simulink model "Vehicle_Performance"  (R2016a)
settings: Solver=ode23s  StartTime=0.0  StopTime=12  FixedStep=0.1  RelTol=1e-3
values from neighbouring files (symbols this model uses):
  a = 0.84    [Vehicle_Performance.mat]
  c = 3100    [Vehicle_Performance.mat]
  d = 30    [Vehicle_Performance.mat]    (also in car_suspension.mat = 0.348888888889)
  e = 2    [Vehicle_Performance.mat]
  gb = 10    [Vehicle_Performance.mat]
  h = 0.65    [Vehicle_Performance.mat]    (also in car_suspension.mat = 353)
  hgr = 0.9    [Vehicle_Performance.mat]
  l = 1.3    [Vehicle_Performance.mat]
  lgr = 3.9    [Vehicle_Performance.mat]
  m = 210    [Vehicle_Performance.mat]
  o = 0    [Vehicle_Performance.mat]
  r = 0.2794    [Vehicle_Performance.mat]    (also in car_suspension.mat = 279.4)
libraries: simulink x3
settings Model: Creator=Lenovo  LastModifiedBy=admin
settings SolverCC: MaxConsecutiveMinStep=100
settings DataIOCC: LimitDataPoints=on  SaveFormat=Array
settings DebuggingCC: AlgebraicLoopMsg=none  ArtificialAlgebraicLoopMsg=none  ParameterPrecisionLossMsg=none
settings HardwareCC: ProdBitPerPointer=32  ProdLargestAtomicFloat=None  ProdIntDivRoundTo=Undefined  ProdEndianess=Unspecified  ProdWordSize=32  ProdHWDeviceType=32-bit Generic
settings ModelReferenceCC: PropagateSignalLabelsOutOfModel=off
settings ConfigComp: CovModelRefEnable=Off  CovSFcnEnable=off
settings ConfigurationSet: Description=SimMechanics 2G

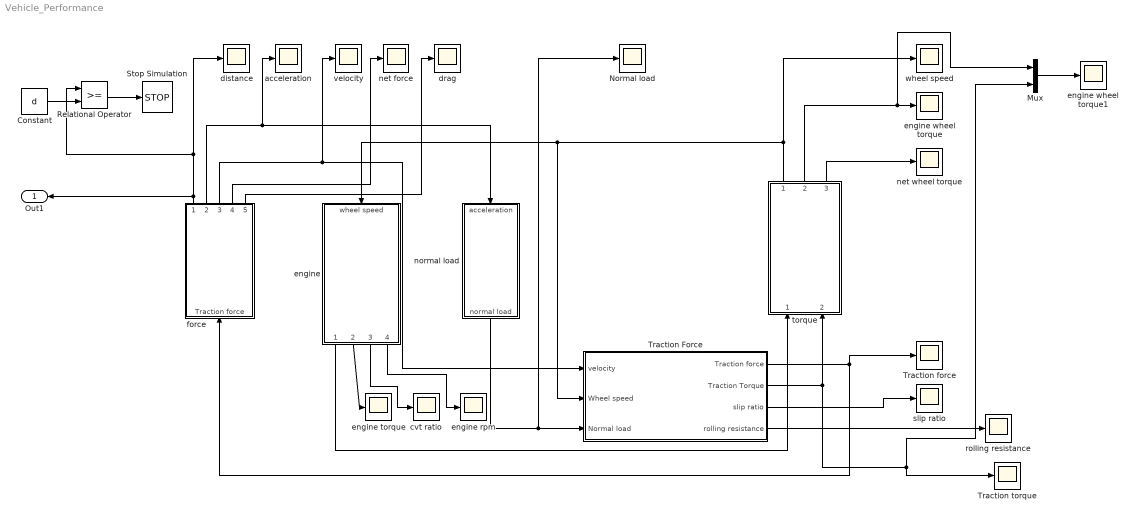
== system Vehicle_Performance ==
  Constant : Constant  Value=d
  Mux : Mux  Inputs=2
  Normal load : Scope
  Relational Operator : RelationalOperator  OutDataTypeStr=boolean
  Stop Simulation : Stop
  Traction Force : Subsystem
  Traction force : Scope
  Traction torque : Scope
  acceleration : Scope
  cvt ratio : Scope
  distance : Scope
  drag : Scope
  "engine " : Subsystem
  engine rpm : Scope
  engine torque : Scope
  engine wheel torque : Scope
  engine wheel torque1 : Scope
  force : Subsystem
  net force : Scope
  net wheel torque : Scope
  normal load : Subsystem
  rolling resistance : Scope
  slip ratio : Scope
  torque : Subsystem
  "velocity " : Scope
  "wheel speed " : Scope
  Out1 : Outport
  wires:
  "engine "/1("wheel torque ") -> torque/1(Wheel torque)
  torque/1("wheel speed ") -> "engine "/1("wheel speed "), Traction Force/2(Wheel speed), "wheel speed "/1
  force/2(acceleration) -> normal load/1(acceleration), acceleration/1
  force/3(Velocity) -> "velocity "/1, Traction Force/1(velocity)
  normal load/1("normal load ") -> Normal load/1, Traction Force/3(Normal load)
  Traction Force/1(Traction force) -> Traction force/1, force/1(Traction force)
  force/1(distance) -> Relational Operator/1, distance/1, Out1/1
  Traction Force/3(slip ratio) -> slip ratio/1
  Traction Force/2(Traction Torque) -> torque/2(Traction torque), Mux/2, Traction torque/1
  torque/3(net wheel torque) -> net wheel torque/1
  force/4(net force) -> net force/1
  force/5(drag force) -> drag/1
  Traction Force/4(rolling resistance) -> rolling resistance/1
  Constant/1 -> Relational Operator/2
  Relational Operator/1 -> Stop Simulation/1
  torque/2(engine wheel torque) -> Mux/1, engine wheel torque/1
  "engine "/2("engine torque  ") -> engine torque/1
  Mux/1 -> engine wheel torque1/1
  "engine "/3(cvt ratio) -> cvt ratio/1
  "engine "/4(engine rpm) -> engine rpm/1

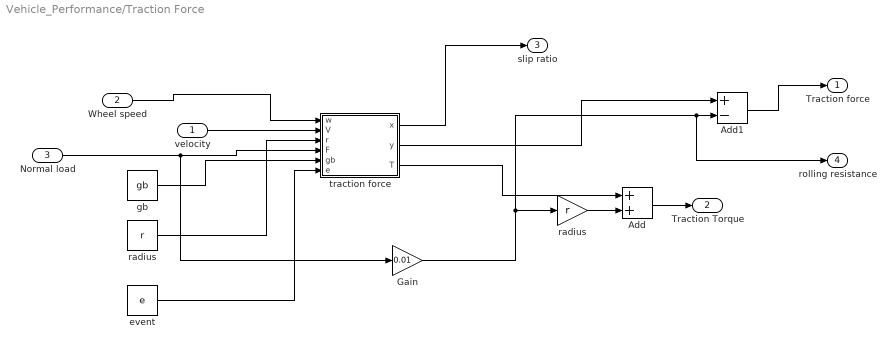
== system Vehicle_Performance/Traction Force ==
  velocity : Inport
  Wheel speed : Inport  Port=2
  Normal load : Inport  Port=3
  Add : Sum
  Add1 : Sum  Inputs=+-
  Gain : Gain  Gain=0.01
  event : Constant  Value=e
  "gb " : Constant  Value=gb
  radius : Gain  Gain=r
  "radius " : Constant  Value=r
  "traction force " : MATLAB Function  TreatAsAtomicUnit=on
  Traction force : Outport
  Traction Torque : Outport  Port=2
  slip ratio : Outport  Port=3
  rolling resistance : Outport  Port=4
  wires:
  velocity/1 -> "traction force "/2(V)
  Wheel speed/1 -> "traction force "/1(w)
  "gb "/1 -> "traction force "/5(gb)
  Normal load/1 -> "traction force "/4(F), Gain/1
  "traction force "/1(x) -> slip ratio/1
  Add/1 -> Traction Torque/1
  "traction force "/3(T) -> Add/1
  Gain/1 -> radius/1, rolling resistance/1, Add1/2
  Add1/1 -> Traction force/1
  "traction force "/2(y) -> Add1/1
  radius/1 -> Add/2
  "radius "/1 -> "traction force "/3(r)
  event/1 -> "traction force "/6(e)

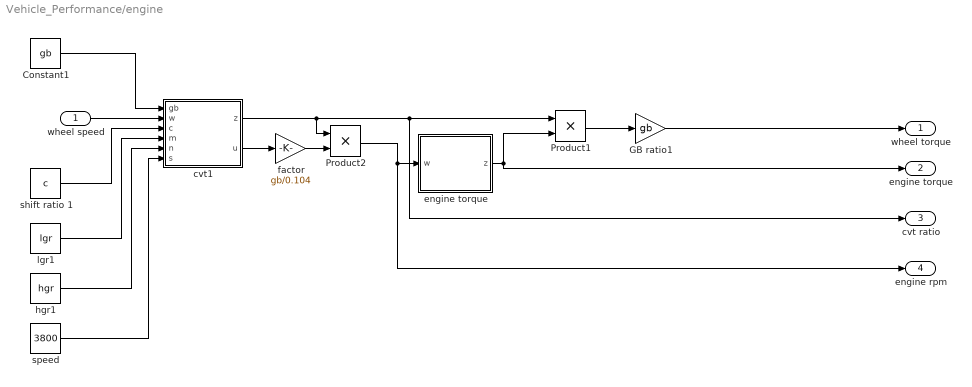
== system Vehicle_Performance/engine  ==
  "wheel speed " : Inport
  Constant1 : Constant  Value=gb
  GB ratio1 : Gain  Gain=gb
  Product1 : Product
  Product2 : Product
  cvt1 : MATLAB Function  TreatAsAtomicUnit=on
  engine torque : MATLAB Function  TreatAsAtomicUnit=on
  factor : Gain  Gain=gb/0.104
  hgr1 : Constant  Value=hgr
  lgr1 : Constant  Value=lgr
  shift ratio 1 : Constant  Value=c
  speed : Constant  Value=3800
  "wheel torque " : Outport
  "engine torque  " : Outport  Port=2
  cvt ratio : Outport  Port=3
  engine rpm : Outport  Port=4
  wires:
  Product1/1 -> GB ratio1/1
  engine torque/1(z) -> "engine torque  "/1, Product1/2
  cvt1/1(z) -> cvt ratio/1, Product1/1, Product2/1
  cvt1/2(u) -> factor/1
  factor/1 -> Product2/2
  Constant1/1 -> cvt1/1(gb)
  shift ratio 1/1 -> cvt1/3(c)
  lgr1/1 -> cvt1/4(m)
  hgr1/1 -> cvt1/5(n)
  speed/1 -> cvt1/6(s)
  Product2/1 -> engine rpm/1, engine torque/1(w)
  GB ratio1/1 -> "wheel torque "/1
  "wheel speed "/1 -> cvt1/2(w)

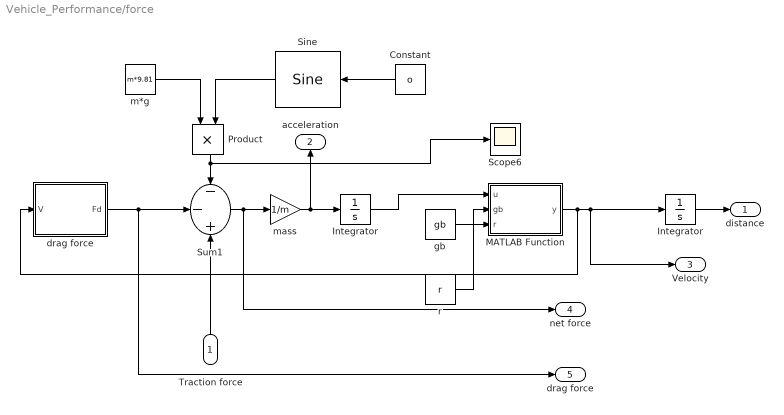
== system Vehicle_Performance/force ==
  Traction force : Inport
  Constant : Constant  Value=o
  "Integrator " : Integrator  LimitOutput=on  UpperSaturationLimit=r*395.2/(gb*hgr)
  "Integrator " : Integrator
  MATLAB Function : MATLAB Function  TreatAsAtomicUnit=on
  Product : Product
  Scope6 : Scope
  Sine : simulink/Lookup Tables/Sine  Formula=sin(2*pi*u)  NumDataPoints=(2^5)+1  OutputWordLength=16  InternalRulePriority=Speed
  Sum1 : Sum  Inputs=--+
  "drag force " : MATLAB Function  TreatAsAtomicUnit=on
  gb : Constant  Value=gb
  m*g : Constant  Value=m*9.81
  mass : Gain  Gain=1/m
  r : Constant  Value=r
  distance : Outport
  acceleration : Outport  Port=2
  Velocity : Outport  Port=3
  net force : Outport  Port=4
  drag force : Outport  Port=5
  wires:
  Sum1/1 -> net force/1, mass/1
  mass/1 -> acceleration/1, "Integrator "/1
  "Integrator "/1 -> distance/1
  Constant/1 -> Sine/1
  m*g/1 -> Product/1
  Sine/1 -> Product/2
  Product/1 -> Sum1/1, Scope6/1
  Traction force/1 -> Sum1/3
  "drag force "/1(Fd) -> Sum1/2, drag force/1
  MATLAB Function/1(y) -> "drag force "/1(V), Velocity/1, "Integrator "/1
  "Integrator "/1 -> MATLAB Function/1(u)
  gb/1 -> MATLAB Function/2(gb)
  r/1 -> MATLAB Function/3(r)

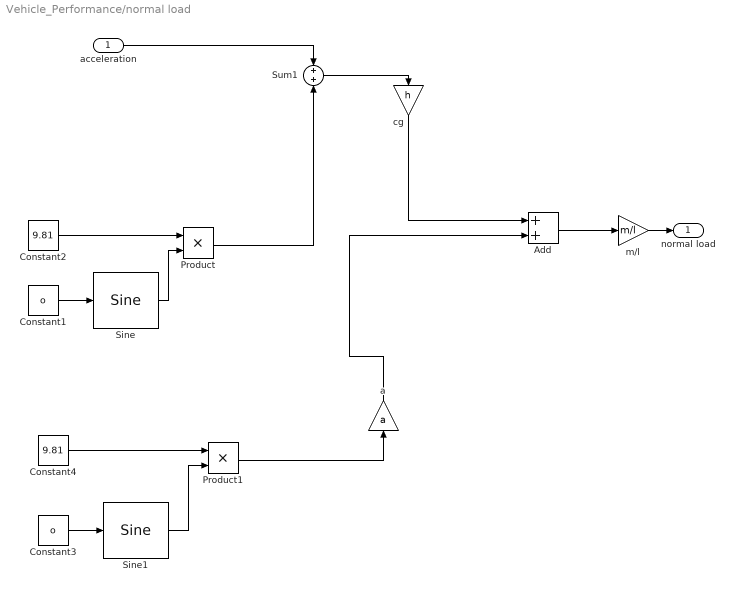
== system Vehicle_Performance/normal load ==
  acceleration : Inport
  Add : Sum
  Constant1 : Constant  Value=o
  Constant2 : Constant  Value=9.81
  Constant3 : Constant  Value=o
  Constant4 : Constant  Value=9.81
  Product : Product
  Product1 : Product
  Sine : simulink/Lookup Tables/Sine  Formula=sin(2*pi*u)  NumDataPoints=(2^5)+1  OutputWordLength=16  InternalRulePriority=Speed
  Sine1 : simulink/Lookup Tables/Sine  Formula=cos(2*pi*u)  NumDataPoints=(2^5)+1  OutputWordLength=16  InternalRulePriority=Speed
  Sum1 : Sum
  a : Gain  Gain=a
  cg : Gain  Gain=h
  m/l : Gain  Gain=m/l
  "normal load " : Outport
  wires:
  m/l/1 -> "normal load "/1
  Constant3/1 -> Sine1/1
  Constant4/1 -> Product1/1
  Sine1/1 -> Product1/2
  Product1/1 -> a/1
  cg/1 -> Add/1
  Constant1/1 -> Sine/1
  Constant2/1 -> Product/1
  Sine/1 -> Product/2
  a/1 -> Add/2
  Add/1 -> m/l/1
  acceleration/1 -> Sum1/1
  Product/1 -> Sum1/2
  Sum1/1 -> cg/1

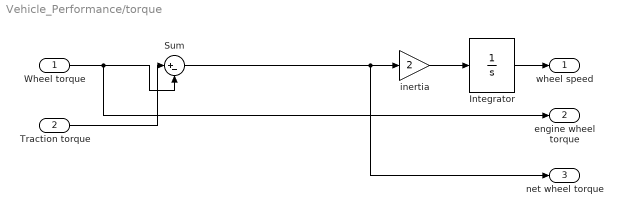
== system Vehicle_Performance/torque ==
  Wheel torque : Inport
  Traction torque : Inport  Port=2
  Integrator : Integrator  InitialCondition=187.2/(lgr*gb)  LimitOutput=on  UpperSaturationLimit=395.2/(gb*hgr)
  Sum : Sum  Inputs=|+-
  inertia : Gain  Gain=2
  "wheel speed " : Outport
  engine wheel torque : Outport  Port=2
  net wheel torque : Outport  Port=3
  wires:
  inertia/1 -> Integrator/1
  Traction torque/1 -> Sum/1
  Wheel torque/1 -> Sum/2, engine wheel torque/1
  Integrator/1 -> "wheel speed "/1
  Sum/1 -> net wheel torque/1, inertia/1

== matlab function Vehicle_Performance/force/MATLAB Function ==
  data: u input; y output; gb input; r input
function y = fcn(u,gb,r)
if u<r*(395.2/(gb*0.9))
    y= u;
else
    y =r*(395.2/(gb*0.9));
end

== matlab function Vehicle_Performance/Traction Force/traction force  ==
  data: x output; w input; y output; V input; r input; F input; T output; gb input; e input
function [x,y,T] = fcn(w,V,r,F,gb,e)
if e == 1
if w<(925.43/gb)
    b = 0.2794*w - V;
    if V > 0.1
    x = b/V;
    else
    x = (2*b/(0.1 + V^2/0.1));
    end
else
    b = 0.2921*(925.43/gb) - V;
    if V > 0.1
    x = b/V;
    else
    x = (2*b/(0.1 + V^2/0.1));
     end
end
y = F*0.75*sin(2.4*atan((7*x-(7*x-atan(7*x)))));
T = y * r;
else
    if w<(925.43/gb)
    b = 0.2794*w - V;
    if V > 0.1
    x = b/V;
    else
    x = (2*b/(0.1 + V^2/0.1));
    end
else
    b = 0.2921*(925.43/gb) - V;
    if V > 0.1
    x = b/V;
    else
    x = (2*b/(0.1 + V^2/0.1));
    end
end
y = F*0.9*sin(1.8*atan((7*x-(7*x-atan(7*x)))));
T = y * r;
end

== matlab function Vehicle_Performance/force/drag force  ==
  data: Fd output; V input
function Fd  = fcn(V)
if V>0
Fd = 0.5*1.225*0.75*0.7*V^2;
else
    Fd= - 0.5*1.225*0.75*0.7*V^2;
end

== matlab function Vehicle_Performance/engine /cvt1 ==
  data: z output; u output; gb input; w input; c input; m input; n input; s input
function [z,u] = fcn(gb,w,c,m,n,s)
 if w < (s*0.104/(gb*n)) 
  if w < (c*0.104/(m*gb))
  z = m;
  else 
  x = [c*0.104/(gb*m) (c*0.104/gb + (s*0.104-0.104*c)/(gb*10))/(m-((m-n)/10)) (c*0.104/gb + 2*(s*0.104-0.104*c)/(gb*10))/(m-2*((m-n)/10)) (c*0.104/gb + 3*(s*0.104-0.104*c)/(gb*10))/(m-3*((m-n)/10)) (c*0.104/gb + 4*(s*0.104-0.104*c)/(gb*10))/(m-4*((m-n)/10)) (c*0.104/gb + 5*(s*0.104-0.104*c)/(gb*10))/(m-5*((m-n)/10)) (c*0.104/gb + 6*(s*0.104-0.104*c)/(gb*10))/(m-6*((m-n)/10)) (c*0.104/gb + 7*(s*0.104-0.104*c)/(gb*10))/(m-7*((m-n)/10)) (c*0.104/gb + 8*(s*0.104-0.104*c)/(gb*10))/(m-8*((m-n)/10)) (c*0.104/gb + 9*(395.2-0.104*c)/(gb*10))/(m-9*((m-n)/10)) ((c*0.104/gb + 9*(395.2-0.104*c)/(gb*10))+395.2/gb)/(2*(m+19*n)/20) s*0.104/(gb*n)];
  y = [m m-((m-n)/10) m-2*((m-n)/10) m-3*((m-n)/10) m-4*((m-n)/10) m-5*((m-n)/10) m-6*((m-n)/10) m-7*((m-n)/10) m-8*((m-n)/10) m-9*((m-n)/10) (m+19*n)/20 n];
  t = polyfit(x,y,5); 
  z = polyval(t,w);
 end
 else
  z = n;
 end
  if w<(395.2/(gb*n))
      u = w;
  else
      u = (395.2/(gb*n));
  end

== matlab function Vehicle_Performance/engine /engine torque ==
  data: w input; z output
function z = fcn(w)
if w<3800
x = [1700 2000 2300 2600 2900 3200 3500 3800];
y = [18 19 19 18 17 17 17 16];
t = polyfit(x,y,6);
z = polyval(t,w);
else
    z = 16
end
